simulink model "untitled"  (R2015b)
settings: Solver=VariableStepAuto  StartTime=0.0  StopTime=2  RelTol=1e-3
values from neighbouring files (symbols this model uses):
  Bf = 3.35e-4    (= 0.000335)    [untitled4.m]
  J = 7.01e-4    (= 0.000701)    [untitled4.m]
  Ke = 0.2960    (= 0.296)    [untitled4.m]
  Kpwm = 384615    [untitled4.m]
  Kt = 0.2939    [untitled4.m]
  La = 2e-3    (= 0.002)    [untitled4.m]
  Ra = 0.92    [untitled4.m]
settings Model: Creator=ovi  LastModifiedBy=ovi

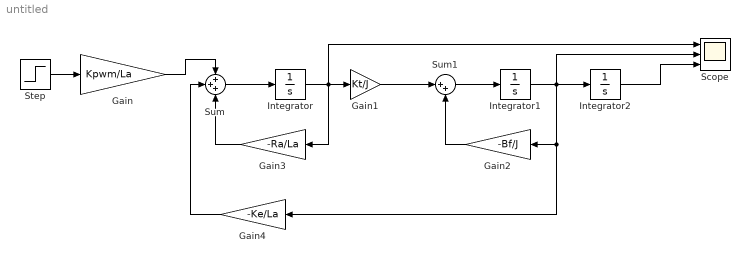
== system untitled ==
  Gain : Gain  Gain=Kpwm/La
  Gain1 : Gain  Gain=Kt/J
  Gain2 : Gain  Gain=-Bf/J
  Gain3 : Gain  Gain=-Ra/La
  Gain4 : Gain  Gain=-Ke/La
  Integrator : Integrator
  Integrator1 : Integrator
  Integrator2 : Integrator
  Scope : Scope  NumInputPorts=3
  Step : Step  SampleTime=0
  Sum : Sum  Inputs=+++
  Sum1 : Sum  Inputs=|++
  wires:
  Step/1 -> Gain/1
  Gain/1 -> Sum/1
  Sum/1 -> Integrator/1
  Integrator/1 -> Gain3/1, Scope/1, Gain1/1
  Gain1/1 -> Sum1/1
  Gain3/1 -> Sum/3
  Sum1/1 -> Integrator1/1
  Integrator1/1 -> Gain4/1, Gain2/1, Scope/2, Integrator2/1
  Integrator2/1 -> Scope/3
  Gain2/1 -> Sum1/2
  Gain4/1 -> Sum/2
